simulink model "reg_track"  (R2014a)
settings: Solver=VariableStepAuto  StartTime=0.0  StopTime=20  RelTol=1e-3
values from neighbouring files (symbols this model uses):
  A = [0 1; -a0 -a1]    [MISO_main.m]    (also in boost_ss.m = [0 -(1-d)/l; (1-d)/c -1/r*c])
  B = [0 ; 1]    [MISO_main.m]    (also in boost_ss.m = [1/l vc_eqm/l; 0 -il_eqm/c])
  C = [b0 b1]    [MISO_main.m]    (also in boost_ss.m = [0 1])
  D = 0    [MISO_main.m]    (also in boost_ss.m = [0])
  Gc = -1/(C*(Ac)^-1*B)    [tracking_MISO.m]
  K = place(A,B,desP)    [Boost_regulator.m]    (also in tracking_MISO.m)
undefined symbols (not defined in the file or in its folder): x0
settings Model: Creator=Bara  LastModifiedBy=Administrator
settings DataIOCC: LimitDataPoints=off  SaveFormat=Dataset
settings OptimizationCC: SimCompilerOptimization=off
settings DebuggingCC: MergeDetectMultiDrivingBlocksExec=error  SolverPrmCheckMsg=none  FrameProcessingCompatibilityMsg=error
settings HardwareCC: ProdBitPerPointer=64  ProdLargestAtomicFloat=Float  ProdIntDivRoundTo=Zero  ProdEndianess=LittleEndian  ProdWordSize=64  ProdHWDeviceType=Intel->x86-64 (Windows64)
settings ModelReferenceCC: PropagateSignalLabelsOutOfModel=on
settings RTWCC: RTWCompilerOptimization=off
settings ConfigComp: CovMetricSettings=dw  CovHtmlReporting=on  CovSaveCumulativeToWorkspaceVar=on  CovSaveSingleToWorkspaceVar=on  CovExternalEMLEnable=off

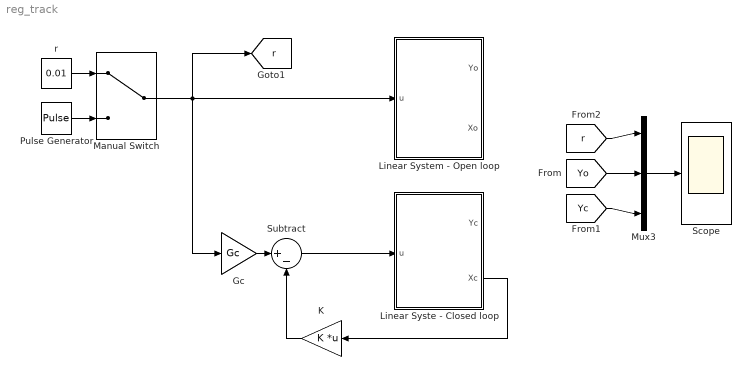
== system reg_track ==
  Gc : Gain  Gain=Gc
  K : Gain  Gain=K  Multiplication=Matrix(K*u) (u vector)
  Linear Syste - Closed loop : Subsystem
  Linear System - Open loop : Subsystem
  Manual Switch : ManualSwitch
  Mux3 : Mux  Inputs=3
  Pulse Generator : DiscretePulseGenerator  PulseType=Time based  Period=10  PulseWidth=50
  Scope : Scope
  Subtract : Sum  Inputs=|+-
  r : Constant  Value=0.01
  tag scope: r=global
  wires:
  Manual Switch/1 -> Linear System - Open loop/1(u), Gc/1, [r]
  Mux3/1 -> Scope/1
  [Yc] -> Mux3/3
  [Yo] -> Mux3/2
  Linear Syste - Closed loop/2(Xc) -> K/1
  K/1 -> Subtract/2
  Subtract/1 -> Linear Syste - Closed loop/1(u)
  Gc/1 -> Subtract/1
  [r] -> Mux3/1
  r/1 -> Manual Switch/1
  Pulse Generator/1 -> Manual Switch/2

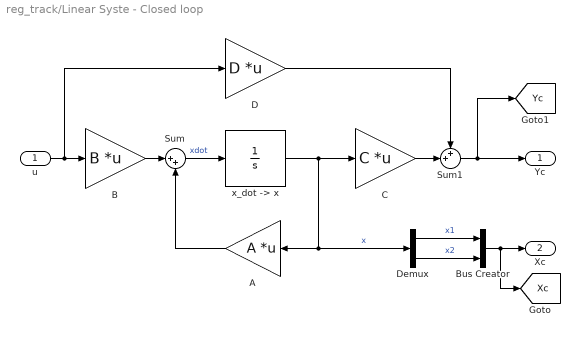
== system reg_track/Linear Syste - Closed loop ==
  u : Inport
  A : Gain  Gain=A  Multiplication=Matrix(K*u) (u vector)
  B : Gain  Gain=B  Multiplication=Matrix(K*u) (u vector)
  Bus Creator : BusCreator  Inputs=2
  C : Gain  Gain=C  Multiplication=Matrix(K*u) (u vector)
  D : Gain  Gain=D  Multiplication=Matrix(K*u) (u vector)
  Demux : Demux  Outputs=2
  Sum : Sum  Inputs=|++
  Sum1 : Sum  Inputs=++|
  "x_dot -> x" : Integrator  InitialCondition=x0
  Yc : Outport
  Xc : Outport  Port=2
  tag scope: Xc=global, Yc=global
  wires:
  Sum/1 -> "x_dot -> x"/1  "xdot"
  "x_dot -> x"/1 -> Demux/1, A/1, C/1  "x"
  A/1 -> Sum/2
  B/1 -> Sum/1
  u/1 -> D/1, B/1
  C/1 -> Sum1/2
  D/1 -> Sum1/1
  Sum1/1 -> [Yc], Yc/1
  Demux/1 -> Bus Creator/1  "x1"
  Demux/2 -> Bus Creator/2  "x2"
  Bus Creator/1 -> Xc/1, [Xc]

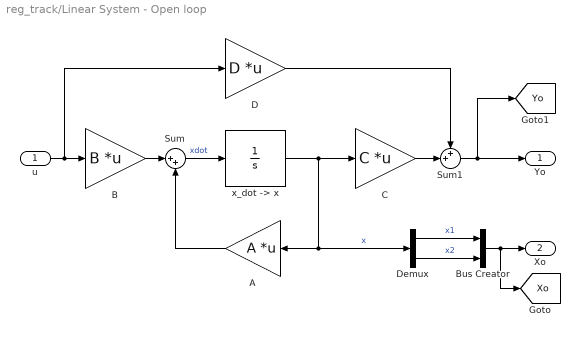
== system reg_track/Linear System - Open loop ==
  u : Inport
  A : Gain  Gain=A  Multiplication=Matrix(K*u) (u vector)
  B : Gain  Gain=B  Multiplication=Matrix(K*u) (u vector)
  Bus Creator : BusCreator  Inputs=2
  C : Gain  Gain=C  Multiplication=Matrix(K*u) (u vector)
  D : Gain  Gain=D  Multiplication=Matrix(K*u) (u vector)
  Demux : Demux  Outputs=2
  Sum : Sum  Inputs=|++
  Sum1 : Sum  Inputs=++|
  "x_dot -> x" : Integrator  InitialCondition=x0
  Yo : Outport
  Xo : Outport  Port=2
  tag scope: Xo=global, Yo=global
  wires:
  Bus Creator/1 -> [Xo], Xo/1
  Demux/2 -> Bus Creator/2  "x2"
  Demux/1 -> Bus Creator/1  "x1"
  Sum1/1 -> Yo/1, [Yo]
  D/1 -> Sum1/1
  C/1 -> Sum1/2
  u/1 -> B/1, D/1
  B/1 -> Sum/1
  A/1 -> Sum/2
  "x_dot -> x"/1 -> C/1, A/1, Demux/1  "x"
  Sum/1 -> "x_dot -> x"/1  "xdot"
